simulink model "stpa_brake_manage_hcs_land"  (R2022a)
settings: Solver=VariableStepAuto  StartTime=0.0  StopTime=10.0  RelTol=1e-3
(part 1 of 2)
settings Model: Creator=E403510  LastModifiedBy=ayj
settings SolverCC: AlgebraicLoopSolver=TrustRegion
settings DataIOCC: ReturnWorkspaceOutputs=off
settings DebuggingCC: UnconnectedInputMsg=warning  UnconnectedOutputMsg=warning  UnconnectedLineMsg=warning  SFMachineParentedDataDiag=warning  ArithmeticOperatorsInVariantConditions=warning
settings SFSimCC: CustomCodeUndefinedFunction=UseInterfaceOnly
settings RTWCC: DLArmComputeVersion=19.05

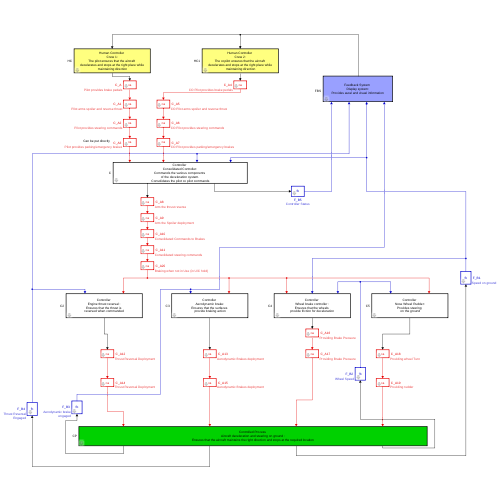
[thumbnail: Simulink's stored preview of the top-level diagram]
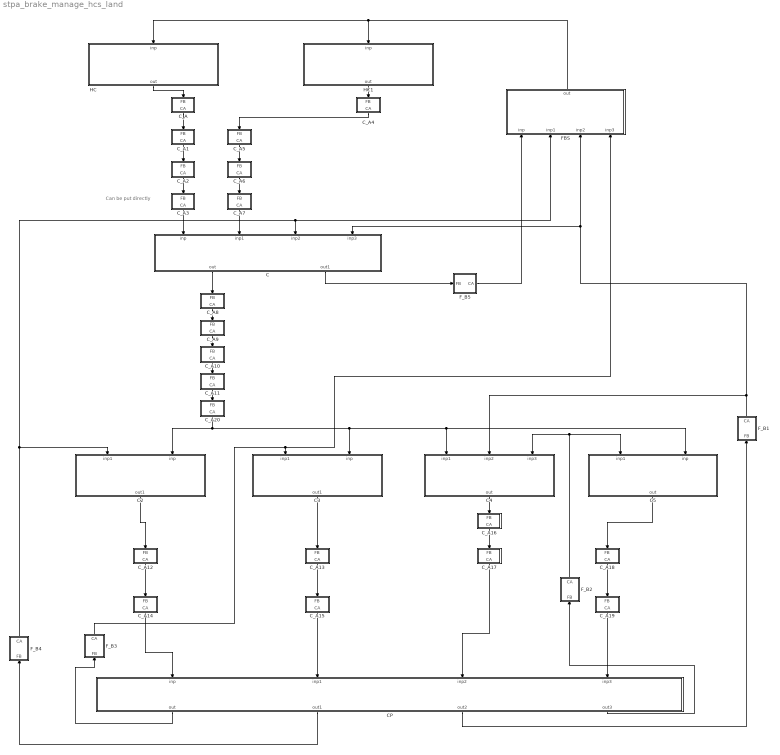
== system stpa_brake_manage_hcs_land ==
  note: Can be put directly
  " FBS" : Subsystem  TreatAsAtomicUnit=on  mask(feedback_system){NAMEFORBLOCK=Display system, DES=Provides aural and visual information}
      mask prompts: NAMEFORBLOCK "Provide a name"; DES "Provide a description of feedback system"
      mask help: Say what this feedback system does
      mask init:
      | set_param(gcb,'LinkStatus', 'none');
      settings: RTWFcnNameOpts=Use subsystem name  RTWFileNameOpts=Use function name
      mask DialogControl Control2 Prompt: ADD Input
      mask DialogControl Control2 Callback:
      | h = add_block('simulink/Sources/In1', [gcb '/inp'], 'MakeNameUnique', 'on');
      | hg = add_block('simulink/Sinks/Terminator', [gcb '/term'], 'MakeNameUnique', 'on');
      | hname = get_param(h,'PortHandles');
      | hgname = get_param(hg,'PortHandles');
      | add_line(gcb, hname.Outport(1), hgname.Inport(1));
      mask DialogControl Control3 Prompt: ADD Output
      mask DialogControl Control3 Callback:
      | h = add_block('simulink/Sinks/Out1', [gcb '/out'], 'MakeNameUnique', 'on');
      | hg = add_block('simulink/Sources/Ground', [gcb '/gnd'], 'MakeNameUnique', 'on');
      | hname = get_param(h,'PortHandles');
      | hgname = get_param(hg,'PortHandles');
      | add_line(gcb, hgname.Outport(1), hname.Inport(1));
      mask DialogControl Control4 Prompt: REM Input
      mask DialogControl Control4 Callback:
      | a=find_system(gcb,'SearchDepth',2,'LookUnderMasks','all','BlockType','Inport');
      | if ~isempty(a)
      | b=get_param(a{1},'PortConnectivity');
      | delete_block(a{1});
      | delete_block(b.DstBlock);
      | delete_line(find_system(gcb, 'SearchDepth',2,'LookUnderMasks','all','FindAll', 'on', 'Type', 'line', 'Connected', 'off'))
      | end
      mask DialogControl Control5 Prompt: REM Output
      mask DialogControl Control5 Callback:
      | a=find_system(gcb,'SearchDepth',2,'LookUnderMasks','all','BlockType','Outport');
      | if ~isempty(a)
      | b=get_param(a{1},'PortConnectivity');
      | delete_block(a{1});
      | delete_block(b.SrcBlock);
      | delete_line(find_system(gcb, 'SearchDepth',2,'LookUnderMasks','all','FindAll', 'on', 'Type', 'line', 'Connected', 'off'))
      | end
      mask Display: disp(['Feedback System \n' NAMEFORBLOCK ':\n' DES])
  C : Subsystem  TreatAsAtomicUnit=on  mask(controller){NAMEFORBLOCK=Consolidated Controller, DES=Commands the various components \n of the deceleration system. \n Consolidates the pilot co pilot commands}
      mask prompts: NAMEFORBLOCK "Provide a name for Block"; DES "Provide a description of Responsibility"
      mask help: Say what this controller does
      mask init:
      | set_param(gcb,'LinkStatus', 'none');
      settings: RTWFcnNameOpts=Use subsystem name  RTWFileNameOpts=Use function name
      mask DialogControl Control2 Prompt: ADD Input
      mask DialogControl Control2 Callback:
      | h = add_block('simulink/Sources/In1', [gcb '/inp'], 'MakeNameUnique', 'on');
      | hg = add_block('simulink/Sinks/Terminator', [gcb '/term'], 'MakeNameUnique', 'on');
      | hname = get_param(h,'PortHandles');
      | hgname = get_param(hg,'PortHandles');
      | add_line(gcb, hname.Outport(1), hgname.Inport(1));
      mask DialogControl Control3 Prompt: ADD Output
      mask DialogControl Control3 Callback:
      | h = add_block('simulink/Sinks/Out1', [gcb '/out'], 'MakeNameUnique', 'on');
      | hg = add_block('simulink/Sources/Ground', [gcb '/gnd'], 'MakeNameUnique', 'on');
      | hname = get_param(h,'PortHandles');
      | hgname = get_param(hg,'PortHandles');
      | add_line(gcb, hgname.Outport(1), hname.Inport(1));
      mask DialogControl Control4 Prompt: REM Input
      mask DialogControl Control4 Callback:
      | a=find_system(gcb,'SearchDepth',2,'LookUnderMasks','all','BlockType','Inport');
      | if ~isempty(a)
      | b=get_param(a{1},'PortConnectivity');
      | delete_block(a{1});
      | delete_block(b.DstBlock);
      | delete_line(find_system(gcb, 'SearchDepth',2,'LookUnderMasks','all','FindAll', 'on', 'Type', 'line', 'Connected', 'off'))
      | end
      mask DialogControl Control5 Prompt: REM Output
      mask DialogControl Control5 Callback:
      | a=find_system(gcb,'SearchDepth',2,'LookUnderMasks','all','BlockType','Outport');
      | if ~isempty(a)
      | b=get_param(a{1},'PortConnectivity');
      | delete_block(a{1});
      | delete_block(b.SrcBlock);
      | delete_line(find_system(gcb, 'SearchDepth',2,'LookUnderMasks','all','FindAll', 'on', 'Type', 'line', 'Connected', 'off'))
      | end
      mask Display: disp(['Controller \n' NAMEFORBLOCK ':\n' DES])
  C2 : Subsystem  TreatAsAtomicUnit=on  mask(controller){NAMEFORBLOCK=Engine thrust reversal, DES=Ensures that the thrust is \n reversed when commanded}
      mask prompts: NAMEFORBLOCK "Provide a name for Block"; DES "Provide a description of Responsibility"
      mask help: Say what this controller does
      mask init:
      | set_param(gcb,'LinkStatus', 'none');
      settings: RTWFcnNameOpts=Use subsystem name  RTWFileNameOpts=Use function name
      mask DialogControl Control2 Prompt: ADD Input
      mask DialogControl Control2 Callback:
      | h = add_block('simulink/Sources/In1', [gcb '/inp'], 'MakeNameUnique', 'on');
      | hg = add_block('simulink/Sinks/Terminator', [gcb '/term'], 'MakeNameUnique', 'on');
      | hname = get_param(h,'PortHandles');
      | hgname = get_param(hg,'PortHandles');
      | add_line(gcb, hname.Outport(1), hgname.Inport(1));
      mask DialogControl Control3 Prompt: ADD Output
      mask DialogControl Control3 Callback:
      | h = add_block('simulink/Sinks/Out1', [gcb '/out'], 'MakeNameUnique', 'on');
      | hg = add_block('simulink/Sources/Ground', [gcb '/gnd'], 'MakeNameUnique', 'on');
      | hname = get_param(h,'PortHandles');
      | hgname = get_param(hg,'PortHandles');
      | add_line(gcb, hgname.Outport(1), hname.Inport(1));
      mask DialogControl Control4 Prompt: REM Input
      mask DialogControl Control4 Callback:
      | a=find_system(gcb,'SearchDepth',2,'LookUnderMasks','all','BlockType','Inport');
      | if ~isempty(a)
      | b=get_param(a{1},'PortConnectivity');
      | delete_block(a{1});
      | delete_block(b.DstBlock);
      | delete_line(find_system(gcb, 'SearchDepth',2,'LookUnderMasks','all','FindAll', 'on', 'Type', 'line', 'Connected', 'off'))
      | end
      mask DialogControl Control5 Prompt: REM Output
      mask DialogControl Control5 Callback:
      | a=find_system(gcb,'SearchDepth',2,'LookUnderMasks','all','BlockType','Outport');
      | if ~isempty(a)
      | b=get_param(a{1},'PortConnectivity');
      | delete_block(a{1});
      | delete_block(b.SrcBlock);
      | delete_line(find_system(gcb, 'SearchDepth',2,'LookUnderMasks','all','FindAll', 'on', 'Type', 'line', 'Connected', 'off'))
      | end
      mask Display: disp(['Controller \n' NAMEFORBLOCK ':\n' DES])
  C3 : Subsystem  TreatAsAtomicUnit=on  mask(controller){NAMEFORBLOCK=Aerodynamic brake, DES=Ensures that the surfaces \n provide braking action}
      mask prompts: NAMEFORBLOCK "Provide a name for Block"; DES "Provide a description of Responsibility"
      mask help: Say what this controller does
      mask init:
      | set_param(gcb,'LinkStatus', 'none');
      settings: RTWFcnNameOpts=Use subsystem name  RTWFileNameOpts=Use function name
      mask DialogControl Control2 Prompt: ADD Input
      mask DialogControl Control2 Callback:
      | h = add_block('simulink/Sources/In1', [gcb '/inp'], 'MakeNameUnique', 'on');
      | hg = add_block('simulink/Sinks/Terminator', [gcb '/term'], 'MakeNameUnique', 'on');
      | hname = get_param(h,'PortHandles');
      | hgname = get_param(hg,'PortHandles');
      | add_line(gcb, hname.Outport(1), hgname.Inport(1));
      mask DialogControl Control3 Prompt: ADD Output
      mask DialogControl Control3 Callback:
      | h = add_block('simulink/Sinks/Out1', [gcb '/out'], 'MakeNameUnique', 'on');
      | hg = add_block('simulink/Sources/Ground', [gcb '/gnd'], 'MakeNameUnique', 'on');
      | hname = get_param(h,'PortHandles');
      | hgname = get_param(hg,'PortHandles');
      | add_line(gcb, hgname.Outport(1), hname.Inport(1));
      mask DialogControl Control4 Prompt: REM Input
      mask DialogControl Control4 Callback:
      | a=find_system(gcb,'SearchDepth',2,'LookUnderMasks','all','BlockType','Inport');
      | if ~isempty(a)
      | b=get_param(a{1},'PortConnectivity');
      | delete_block(a{1});
      | delete_block(b.DstBlock);
      | delete_line(find_system(gcb, 'SearchDepth',2,'LookUnderMasks','all','FindAll', 'on', 'Type', 'line', 'Connected', 'off'))
      | end
      mask DialogControl Control5 Prompt: REM Output
      mask DialogControl Control5 Callback:
      | a=find_system(gcb,'SearchDepth',2,'LookUnderMasks','all','BlockType','Outport');
      | if ~isempty(a)
      | b=get_param(a{1},'PortConnectivity');
      | delete_block(a{1});
      | delete_block(b.SrcBlock);
      | delete_line(find_system(gcb, 'SearchDepth',2,'LookUnderMasks','all','FindAll', 'on', 'Type', 'line', 'Connected', 'off'))
      | end
      mask Display: disp(['Controller \n' NAMEFORBLOCK ':\n' DES])
  C4 : Subsystem  TreatAsAtomicUnit=on  mask(controller){NAMEFORBLOCK=Wheel brake controller, DES=Ensures that the wheels \n provide friction for deceleration}
      mask prompts: NAMEFORBLOCK "Provide a name for Block"; DES "Provide a description of Responsibility"
      mask help: Say what this controller does
      mask init:
      | set_param(gcb,'LinkStatus', 'none');
      settings: RTWFcnNameOpts=Use subsystem name  RTWFileNameOpts=Use function name
      mask DialogControl Control2 Prompt: ADD Input
      mask DialogControl Control2 Callback:
      | h = add_block('simulink/Sources/In1', [gcb '/inp'], 'MakeNameUnique', 'on');
      | hg = add_block('simulink/Sinks/Terminator', [gcb '/term'], 'MakeNameUnique', 'on');
      | hname = get_param(h,'PortHandles');
      | hgname = get_param(hg,'PortHandles');
      | add_line(gcb, hname.Outport(1), hgname.Inport(1));
      mask DialogControl Control3 Prompt: ADD Output
      mask DialogControl Control3 Callback:
      | h = add_block('simulink/Sinks/Out1', [gcb '/out'], 'MakeNameUnique', 'on');
      | hg = add_block('simulink/Sources/Ground', [gcb '/gnd'], 'MakeNameUnique', 'on');
      | hname = get_param(h,'PortHandles');
      | hgname = get_param(hg,'PortHandles');
      | add_line(gcb, hgname.Outport(1), hname.Inport(1));
      mask DialogControl Control4 Prompt: REM Input
      mask DialogControl Control4 Callback:
      | a=find_system(gcb,'SearchDepth',2,'LookUnderMasks','all','BlockType','Inport');
      | if ~isempty(a)
      | b=get_param(a{1},'PortConnectivity');
      | delete_block(a{1});
      | delete_block(b.DstBlock);
      | delete_line(find_system(gcb, 'SearchDepth',2,'LookUnderMasks','all','FindAll', 'on', 'Type', 'line', 'Connected', 'off'))
      | end
      mask DialogControl Control5 Prompt: REM Output
      mask DialogControl Control5 Callback:
      | a=find_system(gcb,'SearchDepth',2,'LookUnderMasks','all','BlockType','Outport');
      | if ~isempty(a)
      | b=get_param(a{1},'PortConnectivity');
      | delete_block(a{1});
      | delete_block(b.SrcBlock);
      | delete_line(find_system(gcb, 'SearchDepth',2,'LookUnderMasks','all','FindAll', 'on', 'Type', 'line', 'Connected', 'off'))
      | end
      mask Display: disp(['Controller \n' NAMEFORBLOCK ':\n' DES])
  C5 : Subsystem  TreatAsAtomicUnit=on  mask(controller){NAMEFORBLOCK=Nose Wheel Rudder, DES=Provides steering \n on the ground}
      mask prompts: NAMEFORBLOCK "Provide a name for Block"; DES "Provide a description of Responsibility"
      mask help: Say what this controller does
      mask init:
      | set_param(gcb,'LinkStatus', 'none');
      settings: RTWFcnNameOpts=Use subsystem name  RTWFileNameOpts=Use function name
      mask DialogControl Control2 Prompt: ADD Input
      mask DialogControl Control2 Callback:
      | h = add_block('simulink/Sources/In1', [gcb '/inp'], 'MakeNameUnique', 'on');
      | hg = add_block('simulink/Sinks/Terminator', [gcb '/term'], 'MakeNameUnique', 'on');
      | hname = get_param(h,'PortHandles');
      | hgname = get_param(hg,'PortHandles');
      | add_line(gcb, hname.Outport(1), hgname.Inport(1));
      mask DialogControl Control3 Prompt: ADD Output
      mask DialogControl Control3 Callback:
      | h = add_block('simulink/Sinks/Out1', [gcb '/out'], 'MakeNameUnique', 'on');
      | hg = add_block('simulink/Sources/Ground', [gcb '/gnd'], 'MakeNameUnique', 'on');
      | hname = get_param(h,'PortHandles');
      | hgname = get_param(hg,'PortHandles');
      | add_line(gcb, hgname.Outport(1), hname.Inport(1));
      mask DialogControl Control4 Prompt: REM Input
      mask DialogControl Control4 Callback:
      | a=find_system(gcb,'SearchDepth',2,'LookUnderMasks','all','BlockType','Inport');
      | if ~isempty(a)
      | b=get_param(a{1},'PortConnectivity');
      | delete_block(a{1});
      | delete_block(b.DstBlock);
      | delete_line(find_system(gcb, 'SearchDepth',2,'LookUnderMasks','all','FindAll', 'on', 'Type', 'line', 'Connected', 'off'))
      | end
      mask DialogControl Control5 Prompt: REM Output
      mask DialogControl Control5 Callback:
      | a=find_system(gcb,'SearchDepth',2,'LookUnderMasks','all','BlockType','Outport');
      | if ~isempty(a)
      | b=get_param(a{1},'PortConnectivity');
      | delete_block(a{1});
      | delete_block(b.SrcBlock);
      | delete_line(find_system(gcb, 'SearchDepth',2,'LookUnderMasks','all','FindAll', 'on', 'Type', 'line', 'Connected', 'off'))
      | end
      mask Display: disp(['Controller \n' NAMEFORBLOCK ':\n' DES])
  CP : Subsystem  TreatAsAtomicUnit=on  mask(controlled_process){NAMEFORBLOCK=Aircraft deceleration and steering on ground, DES=Ensures that the aircraft maintains the right direction and stops at the required location}
      mask prompts: NAMEFORBLOCK "Provide a name for Block"; DES "Provide a description of Responsibility"
      mask help: Say what this controlled process does
      settings: RTWFcnNameOpts=Use subsystem name  RTWFileNameOpts=Use function name
      mask DialogControl Control2 Prompt: ADD Input
      mask DialogControl Control2 Callback:
      | set_param(gcb,'LinkStatus', 'none');
      | h = add_block('simulink/Sources/In1', [gcb '/inp'], 'MakeNameUnique', 'on');
      | hg = add_block('simulink/Sinks/Terminator', [gcb '/term'], 'MakeNameUnique', 'on');
      | hname = get_param(h,'PortHandles');
      | hgname = get_param(hg,'PortHandles');
      | add_line(gcb, hname.Outport(1), hgname.Inport(1));
      mask DialogControl Control3 Prompt: ADD Output
      mask DialogControl Control3 Callback:
      | set_param(gcb,'LinkStatus', 'none');
      | h = add_block('simulink/Sinks/Out1', [gcb '/out'], 'MakeNameUnique', 'on');
      | hg = add_block('simulink/Sources/Ground', [gcb '/gnd'], 'MakeNameUnique', 'on');
      | hname = get_param(h,'PortHandles');
      | hgname = get_param(hg,'PortHandles');
      | add_line(gcb, hgname.Outport(1), hname.Inport(1));
      mask DialogControl Control4 Prompt: REM Input
      mask DialogControl Control4 Callback:
      | set_param(gcb,'LinkStatus', 'none');
      | a=find_system(gcb,'SearchDepth',2,'LookUnderMasks','all','BlockType','Inport');
      | if ~isempty(a)
      | b=get_param(a{1},'PortConnectivity');
      | delete_block(a{1});
      | delete_block(b.DstBlock);
      | delete_line(find_system(gcb, 'SearchDepth',2,'LookUnderMasks','all','FindAll', 'on', 'Type', 'line', 'Connected', 'off'))
      | end
      mask DialogControl Control5 Prompt: REM Output
      mask DialogControl Control5 Callback:
      | set_param(gcb,'LinkStatus', 'none');
      | a=find_system(gcb,'SearchDepth',2,'LookUnderMasks','all','BlockType','Outport');
      | if ~isempty(a)
      | b=get_param(a{1},'PortConnectivity');
      | delete_block(a{1});
      | delete_block(b.SrcBlock);
      | delete_line(find_system(gcb, 'SearchDepth',2,'LookUnderMasks','all','FindAll', 'on', 'Type', 'line', 'Connected', 'off'))
      | end
      mask Display: disp(['Controlled Process \n' NAMEFORBLOCK ':\n' DES])
  C_A : Subsystem  TreatAsAtomicUnit=on  mask(control_action){DES=Pilot provides brake pedals, UCA1=[#H2]Not providing braking on ground, UCA2=[#H4] Providing brake in air, UCA3=[#H2] Providing brake too late on ground, UCA4=[#H2] Stopping brake too soon}
      mask prompts: DES "Provide a description of Control Action"; UCA1 "Not providing causes hazard [link Hazard]"; UCA2 "Providing causes hazard [link Hazard]"; UCA3 "Too early, too late, out of order [link Hazard]"; UCA4 "Stopped too soon, applied too long [link Hazard]"
      mask help:
      | <Source> <Type> <Control Action> <Context> <Link to Hazards>
      | Source = System Above, Type = {provided, not provided ..], Control Action = command
      | from the description, Context = While/When .. Always link to a hazard
      mask init:
      | set_param(gcb,'LinkStatus', 'none');
      settings: AttributesFormatString=%<DES>  RTWFcnNameOpts=Use subsystem name  RTWFileNameOpts=Use function name
      mask Display: disp('ca')
  C_A1 : Subsystem  TreatAsAtomicUnit=on  mask(control_action){DES=Pilot arms spoiler and reverse thrust, UCA1=[#H2] Not arming external system, UCA2=[#H6], UCA3=[#H2] Arms on ground, UCA4=[#H2] Stops the arming process}
      mask prompts: DES "Provide a description of Control Action"; UCA1 "Not providing causes hazard [link Hazard]"; UCA2 "Providing causes hazard [link Hazard]"; UCA3 "Too early, too late, out of order [link Hazard]"; UCA4 "Stopped too soon, applied too long [link Hazard]"
      mask help:
      | <Source> <Type> <Control Action> <Context> <Link to Hazards>
      | Source = System Above, Type = {provided, not provided ..], Control Action = command
      | from the description, Context = While/When .. Always link to a hazard
      mask init:
      | set_param(gcb,'LinkStatus', 'none');
      settings: AttributesFormatString=%<DES>  RTWFcnNameOpts=Use subsystem name  RTWFileNameOpts=Use function name
      mask Display: disp('ca')
  C_A10 : Subsystem  TreatAsAtomicUnit=on  mask(control_action){DES=Consolidated Commands to Brakes, UCA1=[#H2] Not providing commands to brakes on ground (wont stop), UCA2=[#H1] Providing brakes when not commanded, UCA3=[#H2] Commanding brakes too late (wont stop), UCA4=[#H31, #H41] Commanding brakes too long (can skid or lock)}
      mask prompts: DES "Provide a description of Control Action"; UCA1 "Not providing causes hazard [link Hazard]"; UCA2 "Providing causes hazard [link Hazard]"; UCA3 "Too early, too late, out of order [link Hazard]"; UCA4 "Stopped too soon, applied too long [link Hazard]"
      mask help:
      | <Source> <Type> <Control Action> <Context> <Link to Hazards>
      | Source = System Above, Type = {provided, not provided ..], Control Action = command
      | from the description, Context = While/When .. Always link to a hazard
      mask init:
      | set_param(gcb,'LinkStatus', 'none');
      settings: AttributesFormatString=%<DES>  RTWFcnNameOpts=Use subsystem name  RTWFileNameOpts=Use function name
      mask Display: disp('ca')
  C_A11 : Subsystem  TreatAsAtomicUnit=on  mask(control_action){DES=Consolidated steering commands, UCA1=[#H5] Not providing steering on runway, UCA2=[#H51] Providing steering when already on path, UCA3=[#H51] Providing steering out of sync, UCA4=[#H51] Providing steering too long}
      mask prompts: DES "Provide a description of Control Action"; UCA1 "Not providing causes hazard [link Hazard]"; UCA2 "Providing causes hazard [link Hazard]"; UCA3 "Too early, too late, out of order [link Hazard]"; UCA4 "Stopped too soon, applied too long [link Hazard]"
      mask help:
      | <Source> <Type> <Control Action> <Context> <Link to Hazards>
      | Source = System Above, Type = {provided, not provided ..], Control Action = command
      | from the description, Context = While/When .. Always link to a hazard
      mask init:
      | set_param(gcb,'LinkStatus', 'none');
      settings: AttributesFormatString=%<DES>  RTWFcnNameOpts=Use subsystem name  RTWFileNameOpts=Use function name
      mask Display: disp('ca')
  C_A12 : Subsystem  TreatAsAtomicUnit=on  mask(control_action){DES=Thrust Reversal Deployment, UCA1=[#H2] Not providing on touchdown, UCA2=[#H1] Providing in Air, UCA3=[#H4] Providing too late after touchdown, UCA4=[#H2] Providing for a short duration (safe speed not reached)}
      mask prompts: DES "Provide a description of Control Action"; UCA1 "Not providing causes hazard [link Hazard]"; UCA2 "Providing causes hazard [link Hazard]"; UCA3 "Too early, too late, out of order [link Hazard]"; UCA4 "Stopped too soon, applied too long [link Hazard]"
      mask help:
      | <Source> <Type> <Control Action> <Context> <Link to Hazards>
      | Source = System Above, Type = {provided, not provided ..], Control Action = command
      | from the description, Context = While/When .. Always link to a hazard
      mask init:
      | set_param(gcb,'LinkStatus', 'none');
      settings: AttributesFormatString=%<DES>  RTWFcnNameOpts=Use subsystem name  RTWFileNameOpts=Use function name
      mask Display: disp('ca')
  C_A13 : Subsystem  TreatAsAtomicUnit=on  mask(control_action){DES=Aerodynamic Brakes deployment, UCA1=[#H2] Not providing on touchdown, UCA2=[#H1] Providing in Air, UCA3=[#H4] Providing too late after touchdown, UCA4=[#H2] Providing for a short duration (safe speed not reached)}
      mask prompts: DES "Provide a description of Control Action"; UCA1 "Not providing causes hazard [link Hazard]"; UCA2 "Providing causes hazard [link Hazard]"; UCA3 "Too early, too late, out of order [link Hazard]"; UCA4 "Stopped too soon, applied too long [link Hazard]"
      mask help:
      | <Source> <Type> <Control Action> <Context> <Link to Hazards>
      | Source = System Above, Type = {provided, not provided ..], Control Action = command
      | from the description, Context = While/When .. Always link to a hazard
      mask init:
      | set_param(gcb,'LinkStatus', 'none');
      settings: AttributesFormatString=%<DES>  RTWFcnNameOpts=Use subsystem name  RTWFileNameOpts=Use function name
      mask Display: disp('ca')
  C_A14 : Subsystem  TreatAsAtomicUnit=on  mask(control_action){DES=Thrust Reversal Deployment, UCA1=, UCA2=[#H5] Providing unequal, UCA3=, UCA4=}
      mask prompts: DES "Provide a description of Control Action"; UCA1 "Not providing causes hazard [link Hazard]"; UCA2 "Providing causes hazard [link Hazard]"; UCA3 "Too early, too late, out of order [link Hazard]"; UCA4 "Stopped too soon, applied too long [link Hazard]"
      mask help:
      | <Source> <Type> <Control Action> <Context> <Link to Hazards>
      | Source = System Above, Type = {provided, not provided ..], Control Action = command
      | from the description, Context = While/When .. Always link to a hazard
      mask init:
      | set_param(gcb,'LinkStatus', 'none');
      settings: AttributesFormatString=%<DES>  RTWFcnNameOpts=Use subsystem name  RTWFileNameOpts=Use function name
      mask Display: disp('ca')
  C_A15 : Subsystem  TreatAsAtomicUnit=on  mask(control_action){DES=Aerodynamic Brakes deployment, UCA1=, UCA2=[#H5] Providing unequal, UCA3=, UCA4=}
      mask prompts: DES "Provide a description of Control Action"; UCA1 "Not providing causes hazard [link Hazard]"; UCA2 "Providing causes hazard [link Hazard]"; UCA3 "Too early, too late, out of order [link Hazard]"; UCA4 "Stopped too soon, applied too long [link Hazard]"
      mask help:
      | <Source> <Type> <Control Action> <Context> <Link to Hazards>
      | Source = System Above, Type = {provided, not provided ..], Control Action = command
      | from the description, Context = While/When .. Always link to a hazard
      mask init:
      | set_param(gcb,'LinkStatus', 'none');
      settings: AttributesFormatString=%<DES>  RTWFcnNameOpts=Use subsystem name  RTWFileNameOpts=Use function name
      mask Display: disp('ca')
  C_A16 : Subsystem  TreatAsAtomicUnit=on  mask(control_action){DES=Providing Brake Pressure, UCA1=[#H2] Not providing when commanded, UCA2=[#H1] Providing when not commanded, UCA3=[#H4] Providing out of sync, UCA4=[#H31] Applied too long}
      mask prompts: DES "Provide a description of Control Action"; UCA1 "Not providing causes hazard [link Hazard]"; UCA2 "Providing causes hazard [link Hazard]"; UCA3 "Too early, too late, out of order [link Hazard]"; UCA4 "Stopped too soon, applied too long [link Hazard]"
      mask help:
      | <Source> <Type> <Control Action> <Context> <Link to Hazards>
      | Source = System Above, Type = {provided, not provided ..], Control Action = command
      | from the description, Context = While/When .. Always link to a hazard
      mask init:
      | set_param(gcb,'LinkStatus', 'none');
      settings: AttributesFormatString=%<DES>  RTWFcnNameOpts=Use subsystem name  RTWFileNameOpts=Use function name
      mask Display: disp('ca')
  C_A17 : Subsystem  TreatAsAtomicUnit=on  mask(control_action){DES=Providing Brake Pressure, UCA1=, UCA2=[#H41] Providing in air when in use, UCA3=[#H41] Providing before touchdown, UCA4=}
      mask prompts: DES "Provide a description of Control Action"; UCA1 "Not providing causes hazard [link Hazard]"; UCA2 "Providing causes hazard [link Hazard]"; UCA3 "Too early, too late, out of order [link Hazard]"; UCA4 "Stopped too soon, applied too long [link Hazard]"
      mask help:
      | <Source> <Type> <Control Action> <Context> <Link to Hazards>
      | Source = System Above, Type = {provided, not provided ..], Control Action = command
      | from the description, Context = While/When .. Always link to a hazard
      mask init:
      | set_param(gcb,'LinkStatus', 'none');
      settings: AttributesFormatString=%<DES>  RTWFcnNameOpts=Use subsystem name  RTWFileNameOpts=Use function name
      mask Display: disp('ca')
  C_A18 : Subsystem  TreatAsAtomicUnit=on  mask(control_action){DES=Providing wheel Turn, UCA1=[#H51] Not providing when not on center line, UCA2=[#H51] Providing in air (lock), UCA3=[#H51] Providing out of sync, UCA4=[#H51] Applied too long (stuck)}
      mask prompts: DES "Provide a description of Control Action"; UCA1 "Not providing causes hazard [link Hazard]"; UCA2 "Providing causes hazard [link Hazard]"; UCA3 "Too early, too late, out of order [link Hazard]"; UCA4 "Stopped too soon, applied too long [link Hazard]"
      mask help:
      | <Source> <Type> <Control Action> <Context> <Link to Hazards>
      | Source = System Above, Type = {provided, not provided ..], Control Action = command
      | from the description, Context = While/When .. Always link to a hazard
      mask init:
      | set_param(gcb,'LinkStatus', 'none');
      settings: AttributesFormatString=%<DES>  RTWFcnNameOpts=Use subsystem name  RTWFileNameOpts=Use function name
      mask Display: disp('ca')
  C_A19 : Subsystem  TreatAsAtomicUnit=on  mask(control_action){DES=Providing rudder, UCA1=[H51] Not providing when not on center line, UCA2=, UCA3=[#H51] Providing out of sync, UCA4=[#H51] Applied too long}
      mask prompts: DES "Provide a description of Control Action"; UCA1 "Not providing causes hazard [link Hazard]"; UCA2 "Providing causes hazard [link Hazard]"; UCA3 "Too early, too late, out of order [link Hazard]"; UCA4 "Stopped too soon, applied too long [link Hazard]"
      mask help:
      | <Source> <Type> <Control Action> <Context> <Link to Hazards>
      | Source = System Above, Type = {provided, not provided ..], Control Action = command
      | from the description, Context = While/When .. Always link to a hazard
      mask init:
      | set_param(gcb,'LinkStatus', 'none');
      settings: AttributesFormatString=%<DES>  RTWFcnNameOpts=Use subsystem name  RTWFileNameOpts=Use function name
      mask Display: disp('ca')
  C_A2 : Subsystem  TreatAsAtomicUnit=on  mask(control_action){DES=Pilot provides steering commands, UCA1=[#H51] Not providing steering, UCA2=[#H51] Providing steering when not required, UCA3=[#H51] Providing steering when aircraft has already gone off runway, UCA4=[#H51] Providing steering for a long duration cause deviation}
      mask prompts: DES "Provide a description of Control Action"; UCA1 "Not providing causes hazard [link Hazard]"; UCA2 "Providing causes hazard [link Hazard]"; UCA3 "Too early, too late, out of order [link Hazard]"; UCA4 "Stopped too soon, applied too long [link Hazard]"
      mask help:
      | <Source> <Type> <Control Action> <Context> <Link to Hazards>
      | Source = System Above, Type = {provided, not provided ..], Control Action = command
      | from the description, Context = While/When .. Always link to a hazard
      mask init:
      | set_param(gcb,'LinkStatus', 'none');
      settings: AttributesFormatString=%<DES>  RTWFcnNameOpts=Use subsystem name  RTWFileNameOpts=Use function name
      mask Display: disp('ca')
  C_A20 : Subsystem  TreatAsAtomicUnit=on  mask(control_action){DES=Braking when not in Use (in U/C hold), UCA1=[#H61] Not providing brakes when unused, UCA2=[#H1] Providing when in use (not in U/C hold), UCA3=[#H61] Providing out of sync, UCA4=[#H4] Applying even after wheels stop spinning}
      mask prompts: DES "Provide a description of Control Action"; UCA1 "Not providing causes hazard [link Hazard]"; UCA2 "Providing causes hazard [link Hazard]"; UCA3 "Too early, too late, out of order [link Hazard]"; UCA4 "Stopped too soon, applied too long [link Hazard]"
      mask help:
      | <Source> <Type> <Control Action> <Context> <Link to Hazards>
      | Source = System Above, Type = {provided, not provided ..], Control Action = command
      | from the description, Context = While/When .. Always link to a hazard
      mask init:
      | set_param(gcb,'LinkStatus', 'none');
      settings: AttributesFormatString=%<DES>  RTWFcnNameOpts=Use subsystem name  RTWFileNameOpts=Use function name
      mask Display: disp('ca')
  C_A3 : Subsystem  TreatAsAtomicUnit=on  mask(control_action){DES=Pilot provides parking/emergency brakes, UCA1=[#H2] Not providing emergency brake when brakes fail, UCA2=[#H4] Providing emergency brake when brakes are okay - wet runway, UCA3=[#H2] Appying emergency brake brakes when runway wet cause skid, UCA4=[#H5, #H6] Applied emergency brake too long}
      mask prompts: DES "Provide a description of Control Action"; UCA1 "Not providing causes hazard [link Hazard]"; UCA2 "Providing causes hazard [link Hazard]"; UCA3 "Too early, too late, out of order [link Hazard]"; UCA4 "Stopped too soon, applied too long [link Hazard]"
      mask help:
      | <Source> <Type> <Control Action> <Context> <Link to Hazards>
      | Source = System Above, Type = {provided, not provided ..], Control Action = command
      | from the description, Context = While/When .. Always link to a hazard
      mask init:
      | set_param(gcb,'LinkStatus', 'none');
      settings: AttributesFormatString=%<DES>  RTWFcnNameOpts=Use subsystem name  RTWFileNameOpts=Use function name
      mask Display: disp('ca')
  C_A4 : Subsystem  TreatAsAtomicUnit=on  mask(control_action){DES=CO Pilot provides brake pedals, UCA1=[#H2]Not providing braking on ground, UCA2=[#H4] Providing brake in air, UCA3=[#H2] Providing brake too late on ground, UCA4=[#H2] Stopping brake too soon}
      mask prompts: DES "Provide a description of Control Action"; UCA1 "Not providing causes hazard [link Hazard]"; UCA2 "Providing causes hazard [link Hazard]"; UCA3 "Too early, too late, out of order [link Hazard]"; UCA4 "Stopped too soon, applied too long [link Hazard]"
      mask help:
      | <Source> <Type> <Control Action> <Context> <Link to Hazards>
      | Source = System Above, Type = {provided, not provided ..], Control Action = command
      | from the description, Context = While/When .. Always link to a hazard
      mask init:
      | set_param(gcb,'LinkStatus', 'none');
      settings: AttributesFormatString=%<DES>  RTWFcnNameOpts=Use subsystem name  RTWFileNameOpts=Use function name
      mask Display: disp('ca')
  C_A5 : Subsystem  TreatAsAtomicUnit=on  mask(control_action){DES=CO Pilot arms spoiler and reverse thrust, UCA1=[#H2] Not arming external system, UCA2=[#H4], UCA3=[#H2] Arms on ground, UCA4=[#H2] Stops the arming process}
      mask prompts: DES "Provide a description of Control Action"; UCA1 "Not providing causes hazard [link Hazard]"; UCA2 "Providing causes hazard [link Hazard]"; UCA3 "Too early, too late, out of order [link Hazard]"; UCA4 "Stopped too soon, applied too long [link Hazard]"
      mask help:
      | <Source> <Type> <Control Action> <Context> <Link to Hazards>
      | Source = System Above, Type = {provided, not provided ..], Control Action = command
      | from the description, Context = While/When .. Always link to a hazard
      mask init:
      | set_param(gcb,'LinkStatus', 'none');
      settings: AttributesFormatString=%<DES>  RTWFcnNameOpts=Use subsystem name  RTWFileNameOpts=Use function name
      mask Display: disp('ca')
  C_A6 : Subsystem  TreatAsAtomicUnit=on  mask(control_action){DES=CO Pilot provides steering commands, UCA1=[#H51] Not providing steering, UCA2=[#H51] Providing steering when not required, UCA3=[#H51] Providing steering when aircraft has already gone off runway, UCA4=[#H51] Providing steering for a long duration cause deviation}
      mask prompts: DES "Provide a description of Control Action"; UCA1 "Not providing causes hazard [link Hazard]"; UCA2 "Providing causes hazard [link Hazard]"; UCA3 "Too early, too late, out of order [link Hazard]"; UCA4 "Stopped too soon, applied too long [link Hazard]"
      mask help:
      | <Source> <Type> <Control Action> <Context> <Link to Hazards>
      | Source = System Above, Type = {provided, not provided ..], Control Action = command
      | from the description, Context = While/When .. Always link to a hazard
      mask init:
      | set_param(gcb,'LinkStatus', 'none');
      settings: AttributesFormatString=%<DES>  RTWFcnNameOpts=Use subsystem name  RTWFileNameOpts=Use function name
      mask Display: disp('ca')
  C_A7 : Subsystem  TreatAsAtomicUnit=on  mask(control_action){DES=CO Pilot provides parking/emergency brakes, UCA1=[#H2] Not providing emergency brake when brakes fail, UCA2=[#H4] Providing emergency brake when brakes are okay - wet runway, UCA3=[#H2] Appying emergency brake brakes when runway wet cause skid, UCA4=[#H5, #H6] Applied emergency brake too long}
      mask prompts: DES "Provide a description of Control Action"; UCA1 "Not providing causes hazard [link Hazard]"; UCA2 "Providing causes hazard [link Hazard]"; UCA3 "Too early, too late, out of order [link Hazard]"; UCA4 "Stopped too soon, applied too long [link Hazard]"
      mask help:
      | <Source> <Type> <Control Action> <Context> <Link to Hazards>
      | Source = System Above, Type = {provided, not provided ..], Control Action = command
      | from the description, Context = While/When .. Always link to a hazard
      mask init:
      | set_param(gcb,'LinkStatus', 'none');
      settings: AttributesFormatString=%<DES>  RTWFcnNameOpts=Use subsystem name  RTWFileNameOpts=Use function name
      mask Display: disp('ca')
  C_A8 : Subsystem  TreatAsAtomicUnit=on  mask(control_action){DES=Arm the thrust reverse, UCA1=[#H2] Not arming when commanded, UCA2=[#H1] Arming when not commanded, UCA3=[#H2] Arming delayed after commanded, UCA4=[#H2] Not completing Arm in air}
      mask prompts: DES "Provide a description of Control Action"; UCA1 "Not providing causes hazard [link Hazard]"; UCA2 "Providing causes hazard [link Hazard]"; UCA3 "Too early, too late, out of order [link Hazard]"; UCA4 "Stopped too soon, applied too long [link Hazard]"
      mask help:
      | <Source> <Type> <Control Action> <Context> <Link to Hazards>
      | Source = System Above, Type = {provided, not provided ..], Control Action = command
      | from the description, Context = While/When .. Always link to a hazard
      mask init:
      | set_param(gcb,'LinkStatus', 'none');
      settings: AttributesFormatString=%<DES>  RTWFcnNameOpts=Use subsystem name  RTWFileNameOpts=Use function name
      mask Display: disp('ca')
  C_A9 : Subsystem  TreatAsAtomicUnit=on  mask(control_action){DES=Arm the Spoiler deployment, UCA1=[#H2] Not arming when commanded, UCA2=[#H1] Arming when not commanded, UCA3=[#H2] Arming delayed from command, UCA4=[#H2] Not completing Arm in air}
      mask prompts: DES "Provide a description of Control Action"; UCA1 "Not providing causes hazard [link Hazard]"; UCA2 "Providing causes hazard [link Hazard]"; UCA3 "Too early, too late, out of order [link Hazard]"; UCA4 "Stopped too soon, applied too long [link Hazard]"
      mask help:
      | <Source> <Type> <Control Action> <Context> <Link to Hazards>
      | Source = System Above, Type = {provided, not provided ..], Control Action = command
      | from the description, Context = While/When .. Always link to a hazard
      mask init:
      | set_param(gcb,'LinkStatus', 'none');
      settings: AttributesFormatString=%<DES>  RTWFcnNameOpts=Use subsystem name  RTWFileNameOpts=Use function name
      mask Display: disp('ca')
  F_B1 : Subsystem  TreatAsAtomicUnit=on  mask(feedback){DES=Speed on ground}
      mask prompts: DES "Provide a description"
      mask help: Say what this feeds back from the system
      mask init:
      | set_param(gcb,'LinkStatus', 'none');
      settings: AttributesFormatString=%<DES>  RTWFcnNameOpts=Use subsystem name  RTWFileNameOpts=Use function name
      mask Display: disp('fb')
  F_B2 : Subsystem  TreatAsAtomicUnit=on  mask(feedback){DES=Wheel Speed}
      mask prompts: DES "Provide a description"
      mask help: Say what this feeds back from the system
      mask init:
      | set_param(gcb,'LinkStatus', 'none');
      settings: AttributesFormatString=%<DES>  RTWFcnNameOpts=Use subsystem name  RTWFileNameOpts=Use function name
      mask Display: disp('fb')
  F_B3 : Subsystem  TreatAsAtomicUnit=on  mask(feedback){DES=Aerodynamic brake\n engaged}
      mask prompts: DES "Provide a description"
      mask help: Say what this feeds back from the system
      mask init:
      | set_param(gcb,'LinkStatus', 'none');
      settings: AttributesFormatString=%<DES>  RTWFcnNameOpts=Use subsystem name  RTWFileNameOpts=Use function name
      mask Display: disp('fb')
  F_B4 : Subsystem  TreatAsAtomicUnit=on  mask(feedback){DES=Thrust Reversal\n Engaged}
      mask prompts: DES "Provide a description"
      mask help: Say what this feeds back from the system
      mask init:
      | set_param(gcb,'LinkStatus', 'none');
      settings: AttributesFormatString=%<DES>  RTWFcnNameOpts=Use subsystem name  RTWFileNameOpts=Use function name
      mask Display: disp('fb')
  F_B5 : Subsystem  TreatAsAtomicUnit=on  mask(feedback){DES=Controller Status}
      mask prompts: DES "Provide a description"
      mask help: Say what this feeds back from the system
      mask init:
      | set_param(gcb,'LinkStatus', 'none');
      settings: AttributesFormatString=%<DES>  RTWFcnNameOpts=Use subsystem name  RTWFileNameOpts=Use function name
      mask Display: disp('fb')
  HC : Subsystem  TreatAsAtomicUnit=on  mask(human_controller){NAMEFORBLOCK=Crew 1, DES=The pilot ensures that the aircraft \n decelerates and stops at the right place while \n maintaining direction}
      mask prompts: NAMEFORBLOCK "Provide a name for Block"; DES "Provide a description of Responsibility"
      mask help: Say what this human controller does
      mask init:
      | set_param(gcb,'LinkStatus','none')
      settings: RTWFcnNameOpts=Use subsystem name  RTWFileNameOpts=Use function name
      mask DialogControl Control2 Prompt: ADD Input
      mask DialogControl Control2 Callback:
      | h = add_block('simulink/Sources/In1', [gcb '/inp'], 'MakeNameUnique', 'on');
      | hg = add_block('simulink/Sinks/Terminator', [gcb '/term'], 'MakeNameUnique', 'on');
      | hname = get_param(h,'PortHandles');
      | hgname = get_param(hg,'PortHandles');
      | add_line(gcb, hname.Outport(1), hgname.Inport(1));
      mask DialogControl Control3 Prompt: ADD Output
      mask DialogControl Control3 Callback:
      | h = add_block('simulink/Sinks/Out1', [gcb '/out'], 'MakeNameUnique', 'on');
      | hg = add_block('simulink/Sources/Ground', [gcb '/gnd'], 'MakeNameUnique', 'on');
      | hname = get_param(h,'PortHandles');
      | hgname = get_param(hg,'PortHandles');
      | add_line(gcb, hgname.Outport(1), hname.Inport(1));
      mask DialogControl Control4 Prompt: REM Input
      mask DialogControl Control4 Callback:
      | a=find_system(gcb,'SearchDepth',2,'LookUnderMasks','all','BlockType','Inport');
      | if ~isempty(a)
      | b=get_param(a{1},'PortConnectivity');
      | delete_block(a{1});
      | delete_block(b.DstBlock);
      | delete_line(find_system(gcb, 'SearchDepth',2,'LookUnderMasks','all','FindAll', 'on', 'Type', 'line', 'Connected', 'off'))
      | end
      mask DialogControl Control5 Prompt: REM Output
      mask DialogControl Control5 Callback:
      | a=find_system(gcb,'SearchDepth',2,'LookUnderMasks','all','BlockType','Outport');
      | if ~isempty(a)
      | b=get_param(a{1},'PortConnectivity');
      | delete_block(a{1});
      | delete_block(b.SrcBlock);
      | delete_line(find_system(gcb, 'SearchDepth',2,'LookUnderMasks','all','FindAll', 'on', 'Type', 'line', 'Connected', 'off'))
      | end
      mask Display: disp(['Human Controller \n' NAMEFORBLOCK ':\n' DES])
  HC1 : Subsystem  TreatAsAtomicUnit=on  mask(human_controller){NAMEFORBLOCK=Crew 2, DES=The copilot ensures that the aircraft \n decelerates and stops at the right place while \n maintaining direction}
      mask prompts: NAMEFORBLOCK "Provide a name for Block"; DES "Provide a description of Responsibility"
      mask help: Say what this human controller does
      mask init:
      | set_param(gcb,'LinkStatus','none')
      settings: RTWFcnNameOpts=Use subsystem name  RTWFileNameOpts=Use function name
      mask DialogControl Control2 Prompt: ADD Input
      mask DialogControl Control2 Callback:
      | h = add_block('simulink/Sources/In1', [gcb '/inp'], 'MakeNameUnique', 'on');
      | hg = add_block('simulink/Sinks/Terminator', [gcb '/term'], 'MakeNameUnique', 'on');
      | hname = get_param(h,'PortHandles');
      | hgname = get_param(hg,'PortHandles');
      | add_line(gcb, hname.Outport(1), hgname.Inport(1));
      mask DialogControl Control3 Prompt: ADD Output
      mask DialogControl Control3 Callback:
      | h = add_block('simulink/Sinks/Out1', [gcb '/out'], 'MakeNameUnique', 'on');
      | hg = add_block('simulink/Sources/Ground', [gcb '/gnd'], 'MakeNameUnique', 'on');
      | hname = get_param(h,'PortHandles');
      | hgname = get_param(hg,'PortHandles');
      | add_line(gcb, hgname.Outport(1), hname.Inport(1));
      mask DialogControl Control4 Prompt: REM Input
      mask DialogControl Control4 Callback:
      | a=find_system(gcb,'SearchDepth',2,'LookUnderMasks','all','BlockType','Inport');
      | if ~isempty(a)
      | b=get_param(a{1},'PortConnectivity');
      | delete_block(a{1});
      | delete_block(b.DstBlock);
      | delete_line(find_system(gcb, 'SearchDepth',2,'LookUnderMasks','all','FindAll', 'on', 'Type', 'line', 'Connected', 'off'))
      | end
      mask DialogControl Control5 Prompt: REM Output
      mask DialogControl Control5 Callback:
      | a=find_system(gcb,'SearchDepth',2,'LookUnderMasks','all','BlockType','Outport');
      | if ~isempty(a)
      | b=get_param(a{1},'PortConnectivity');
      | delete_block(a{1});
      | delete_block(b.SrcBlock);
      | delete_line(find_system(gcb, 'SearchDepth',2,'LookUnderMasks','all','FindAll', 'on', 'Type', 'line', 'Connected', 'off'))
      | end
      mask Display: disp(['Human Controller \n' NAMEFORBLOCK ':\n' DES])
  wires:
  HC/1(out) -> C_A/1(FB)
  HC1/1(out) -> C_A4/1(FB)
  C/1(out) -> C_A8/1(FB)
  C2/1(out1) -> C_A12/1(FB)
  C5/1(out) -> C_A18/1(FB)
  " FBS"/1(out) -> HC1/1(inp), HC/1(inp)
  C/2(out1) -> F_B5/1(FB)
  F_B4/1(CA) -> C2/1(inp1), C/3(inp2), " FBS"/2(inp1)
  CP/3(out2) -> F_B1/1(FB)
  F_B1/1(CA) -> C4/2(inp2), C/4(inp3), " FBS"/3(inp2)
  C_A/1(CA) -> C_A1/1(FB)
  C_A1/1(CA) -> C_A2/1(FB)
  C_A2/1(CA) -> C_A3/1(FB)
  C_A3/1(CA) -> C/1(inp)
  C_A4/1(CA) -> C_A5/1(FB)
  C_A5/1(CA) -> C_A6/1(FB)
  C_A6/1(CA) -> C_A7/1(FB)
  C_A7/1(CA) -> C/2(inp1)
  C_A8/1(CA) -> C_A9/1(FB)
  C_A9/1(CA) -> C_A10/1(FB)
  C_A10/1(CA) -> C_A11/1(FB)
  C_A11/1(CA) -> C_A20/1(FB)
  C_A12/1(CA) -> C_A14/1(FB)
  C_A13/1(CA) -> C_A15/1(FB)
  C_A14/1(CA) -> CP/1(inp)
  C_A15/1(CA) -> CP/2(inp1)
  C4/1(out) -> C_A16/1(FB)
  C_A16/1(CA) -> C_A17/1(FB)
  C_A17/1(CA) -> CP/3(inp2)
  C_A18/1(CA) -> C_A19/1(FB)
  C_A19/1(CA) -> CP/4(inp3)
  F_B2/1(CA) -> C5/1(inp1), C4/3(inp3)
  CP/4(out3) -> F_B2/1(FB)
  C_A20/1(CA) -> C2/2(inp), C3/2(inp), C5/2(inp), C4/1(inp1)
  CP/1(out) -> F_B3/1(FB)
  F_B3/1(CA) -> " FBS"/4(inp3), C3/1(inp1)
  C3/1(out1) -> C_A13/1(FB)
  CP/2(out1) -> F_B4/1(FB)
  F_B5/1(CA) -> " FBS"/1(inp)

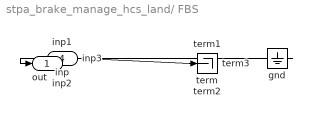
== system stpa_brake_manage_hcs_land/ FBS ==
  inp : Inport
  inp1 : Inport  Port=2
  inp2 : Inport  Port=3
  inp3 : Inport  Port=4
  gnd : Ground
  term{,1..3} (4 alike) : Terminator
  out : Outport
  wires:
  inp/1 -> term/1
  gnd/1 -> out/1
  inp1/1 -> term1/1
  inp2/1 -> term2/1
  inp3/1 -> term3/1

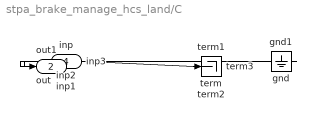
== system stpa_brake_manage_hcs_land/C ==
  inp : Inport
  inp1 : Inport  Port=2
  inp2 : Inport  Port=3
  inp3 : Inport  Port=4
  gnd : Ground
  gnd1 : Ground
  term{,1..3} (4 alike) : Terminator
  out : Outport  VectorParamsAs1DForOutWhenUnconnected=off
  out1 : Outport  Port=2
  wires:
  gnd/1 -> out/1
  inp/1 -> term/1
  inp1/1 -> term1/1
  gnd1/1 -> out1/1
  inp2/1 -> term2/1
  inp3/1 -> term3/1

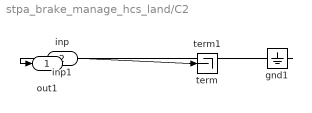
== system stpa_brake_manage_hcs_land/C2 ==
  inp1 : Inport
  inp : Inport  Port=2
  gnd1 : Ground
  term : Terminator
  term1 : Terminator
  out1 : Outport
  wires:
  inp1/1 -> term1/1
  gnd1/1 -> out1/1
  inp/1 -> term/1

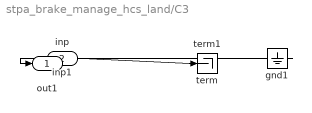
== system stpa_brake_manage_hcs_land/C3 ==
  inp1 : Inport
  inp : Inport  Port=2
  gnd1 : Ground
  term : Terminator
  term1 : Terminator
  out1 : Outport
  wires:
  inp1/1 -> term1/1
  gnd1/1 -> out1/1
  inp/1 -> term/1

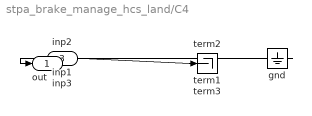
== system stpa_brake_manage_hcs_land/C4 ==
  inp1 : Inport
  inp2 : Inport  Port=2
  inp3 : Inport  Port=3
  gnd : Ground
  term1 : Terminator
  term2 : Terminator
  term3 : Terminator
  out : Outport  VectorParamsAs1DForOutWhenUnconnected=off
  wires:
  inp1/1 -> term1/1
  gnd/1 -> out/1
  inp2/1 -> term2/1
  inp3/1 -> term3/1

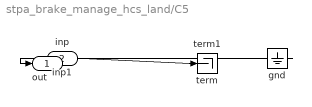
== system stpa_brake_manage_hcs_land/C5 ==
  inp1 : Inport
  inp : Inport  Port=2
  gnd : Ground
  term : Terminator
  term1 : Terminator
  out : Outport  VectorParamsAs1DForOutWhenUnconnected=off
  wires:
  gnd/1 -> out/1
  inp1/1 -> term1/1
  inp/1 -> term/1

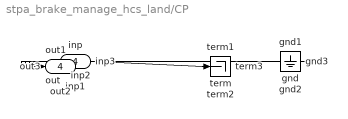
== system stpa_brake_manage_hcs_land/CP ==
  inp : Inport
  inp1 : Inport  Port=2
  inp2 : Inport  Port=3
  inp3 : Inport  Port=4
  gnd{,1..3} (4 alike) : Ground
  term{,1..3} (4 alike) : Terminator
  out : Outport  VectorParamsAs1DForOutWhenUnconnected=off
  out1 : Outport  Port=2
  out2 : Outport  Port=3
  out3 : Outport  Port=4
  wires:
  inp/1 -> term/1
  gnd/1 -> out/1
  inp1/1 -> term1/1
  inp2/1 -> term2/1
  inp3/1 -> term3/1
  gnd1/1 -> out1/1
  gnd2/1 -> out2/1
  gnd3/1 -> out3/1

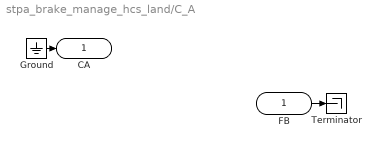
== system stpa_brake_manage_hcs_land/C_A ==
  FB : Inport
      mask Display:
      | plot([0 60-10],[0 0]);
      | plot([0 0],[0 16]);
      | plot([0 60-10],[16 16]);
      | plot([60-10 60],[16 8]);
      | plot([60-10 60],[0 8]);
  Ground : Ground
  Terminator : Terminator
  CA : Outport
      mask Display:
      | plot([10 65],[0 0]);
      | plot([65-1 65-1],[0 16]);
      | plot([10 65],[16 16]);
      | plot([0 10],[8 16]);
      | plot([0 10],[8 0]);
  wires:
  FB/1 -> Terminator/1
  Ground/1 -> CA/1

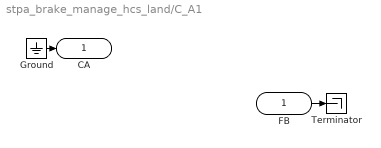
== system stpa_brake_manage_hcs_land/C_A1 ==
  FB : Inport
      mask Display:
      | plot([0 60-10],[0 0]);
      | plot([0 0],[0 16]);
      | plot([0 60-10],[16 16]);
      | plot([60-10 60],[16 8]);
      | plot([60-10 60],[0 8]);
  Ground : Ground
  Terminator : Terminator
  CA : Outport
      mask Display:
      | plot([10 65],[0 0]);
      | plot([65-1 65-1],[0 16]);
      | plot([10 65],[16 16]);
      | plot([0 10],[8 16]);
      | plot([0 10],[8 0]);
  wires:
  Ground/1 -> CA/1
  FB/1 -> Terminator/1

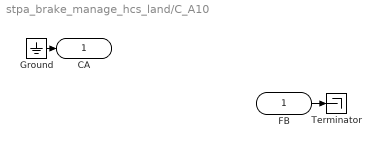
== system stpa_brake_manage_hcs_land/C_A10 ==
  FB : Inport
      mask Display:
      | plot([0 60-10],[0 0]);
      | plot([0 0],[0 16]);
      | plot([0 60-10],[16 16]);
      | plot([60-10 60],[16 8]);
      | plot([60-10 60],[0 8]);
  Ground : Ground
  Terminator : Terminator
  CA : Outport
      mask Display:
      | plot([10 65],[0 0]);
      | plot([65-1 65-1],[0 16]);
      | plot([10 65],[16 16]);
      | plot([0 10],[8 16]);
      | plot([0 10],[8 0]);
  wires:
  Ground/1 -> CA/1
  FB/1 -> Terminator/1

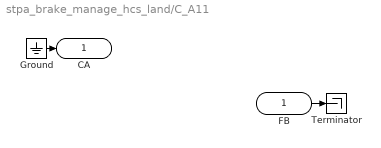
== system stpa_brake_manage_hcs_land/C_A11 ==
  FB : Inport
      mask Display:
      | plot([0 60-10],[0 0]);
      | plot([0 0],[0 16]);
      | plot([0 60-10],[16 16]);
      | plot([60-10 60],[16 8]);
      | plot([60-10 60],[0 8]);
  Ground : Ground
  Terminator : Terminator
  CA : Outport
      mask Display:
      | plot([10 65],[0 0]);
      | plot([65-1 65-1],[0 16]);
      | plot([10 65],[16 16]);
      | plot([0 10],[8 16]);
      | plot([0 10],[8 0]);
  wires:
  FB/1 -> Terminator/1
  Ground/1 -> CA/1
